simulink model "sampleModel257"  (R2021b)
settings: Solver=VariableStepAuto  StartTime=0.0  StopTime=10.0  RelTol=1e-3
undefined symbols (not defined in the file or in its folder): DiscIntNeverNeededParam, Newton, Raphson
libraries: simulink x16, slpidlib x1
settings Model: Creator=user  LastModifiedBy=user

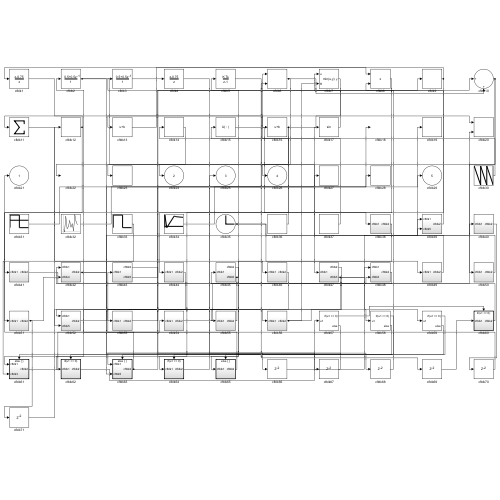
[thumbnail: Simulink's stored preview of the top-level diagram]
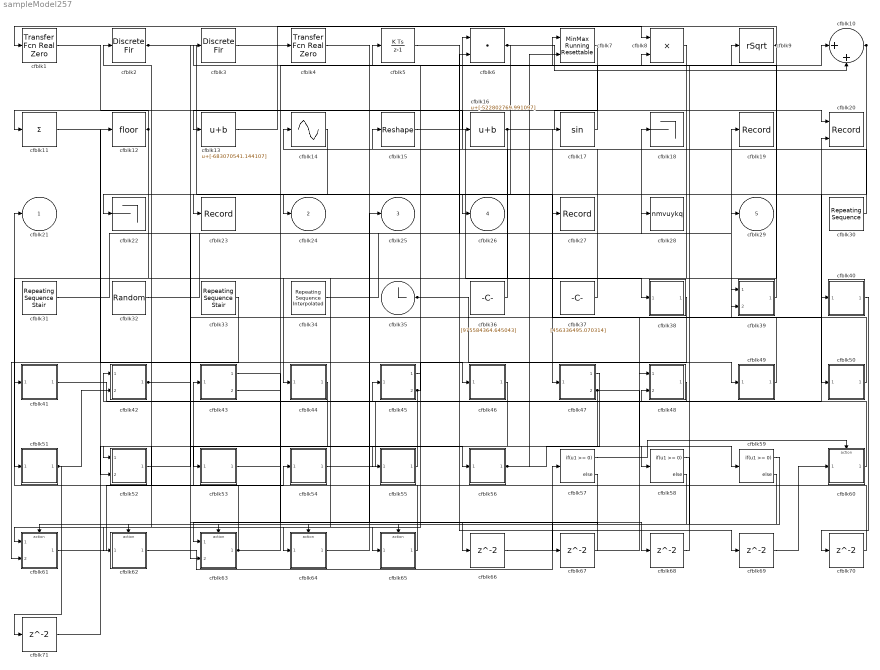
== system sampleModel257 ==
  cfblk1 : simulink/Discrete/Transfer Fcn Real Zero  ZeroZ=0.75  ICPrevInput=0.0  DoSatur=off
      settings: SourceProductBaseCode=SL
  cfblk10 : Sum  Inputs=|++
  cfblk11 : Sum  Inputs=+
  cfblk12 : Rounding
  cfblk13 : Bias  Bias=[-683070541.144107]
  cfblk14 : Sin  TimeSource=Use external signal  SampleTime=0
  cfblk15 : Reshape
  cfblk16 : Bias  Bias=[-522802769.991097]
  cfblk17 : Trigonometry
  cfblk18 : Terminator
  cfblk19 : Record  FileSettingsInternal="{\"entries\":[{\"content\":{\"excelSettings\":{\"content\":{},\"type\":\"Streamout.ExcelSettings\"}},\"type\":\"Streamout.FileSettingStorage\",\"uuid\":\"2ab1578b-86c7-4f25-b23b-f8d6f15a5c50\"}],\"packageUris\":[\"http://schema.mathworks.com/mf0/streamout_blocks/R2020a\"],\"version\":\"1.0\"}"  SignalsInternal="{\"entries\":[{\"content\":{\"signals\":[{\"content\":{\"blockPath\":[\"sampleModel257/cfblk19\"],\"channel\":[],\"dimensions\":[1],\"domain\":\"sampleModel257/cfblk19\",\"lineColor\":\"#fe330a\",\"plots\":[1],\"port\":1,\"sid\":[\"\"],\"signalID\":10619,\"signalName\":\"cfblk32\"},\"type\":\"RecordBlkView.Signal\",\"uuid\":\"c116c59d-c383-4a62-b9dd-bef188b6a92c\"}]},\"type\":\"RecordBlkView.InputSignals\",\"uuid\":\"59890f28-61aa-4252-838f-816ff403dd3c\"}],\"packageUris\":[\"http://schema.mathworks.com/mf0/streamout_blocks/R2020a\"],\"version\":\"1.0\"}"  VisualizationBindings="{\"sparklinesplugin\":{\"info\":[{\"bindingParametersList\":[],\"subplotID\":1}]}}"
  cfblk2 : DiscreteFir  SampleTime=1
  cfblk20 : Record  FileSettingsInternal="{\"entries\":[{\"content\":{\"excelSettings\":{\"content\":{},\"type\":\"Streamout.ExcelSettings\"}},\"type\":\"Streamout.FileSettingStorage\",\"uuid\":\"ddf2c5f0-8deb-4ac6-b6ac-07b526f580c7\"}],\"packageUris\":[\"http://schema.mathworks.com/mf0/streamout_blocks/R2020a\"],\"version\":\"1.0\"}"  Layout=[1 1]  SignalsInternal="{\"entries\":[{\"content\":{\"signals\":[{\"content\":{\"blockPath\":[\"sampleModel257/cfblk20\"],\"channel\":[],\"dimensions\":[1],\"domain\":\"sampleModel257/cfblk20\",\"lineColor\":\"#a2142f\",\"plots\":[1],\"port\":1,\"sid\":[\"\"],\"signalID\":10603,\"signalName\":\"cfblk16\"},\"type\":\"RecordBlkView.Signal\",\"uuid\":\"a0e00e2b-60e6-43d2-9d8d-836ea06b8f3f\"},{\"content\":{\"blockPath\":[\"sampleModel257/cfblk20\"],\"channel\":[],\"dimensions\":[1],\"domain\":\"sampleModel257/cfblk20\",\"lineColor\":\"#139fff\",\"plots\":[1],\"port\":2,\"sid\":[\"\"],\"signalID\":10607,\"signalName\":\"cfblk54\"},\"type\":\"RecordBlkView.Signal\",\"uuid\":\"187d8806-91fd-4e25-8316-ecd599589666\"}]},\"type\":\"RecordBlkView.InputSignals\",\"uuid\":\"124e2f7b-5629-4b4f-94f6-d1d15d40ce0e\"}],\"packageUris\":[\"http://schema.mathworks.com/mf0/streamout_blocks/R2020a\"],\"version\":\"1.0\"}"  VisualizationBindings="{\"xyplotplugin\":{\"info\":[{\"series\":[{\"bindingParametersList\":[{\"parameter\":\"X-Axis\",\"signalID\":10603,\"signalName\":\"cfblk16\"},{\"parameter\":\"Y-Axis\",\"signalID\":10607,\"signalName\":\"cfblk54\"}],\"seriesID\":16544}],\"subplotID\":1}]}}"  CompatibilityTag=XY
  cfblk22 : Terminator
  cfblk23 : Record  FileSettingsInternal="{\"entries\":[{\"content\":{\"excelSettings\":{\"content\":{},\"type\":\"Streamout.ExcelSettings\"}},\"type\":\"Streamout.FileSettingStorage\",\"uuid\":\"70e21285-8622-4f4c-8864-935dd75f7605\"}],\"packageUris\":[\"http://schema.mathworks.com/mf0/streamout_blocks/R2020a\"],\"version\":\"1.0\"}"  SignalsInternal="{\"entries\":[{\"content\":{\"signals\":[{\"content\":{\"blockPath\":[\"sampleModel257/cfblk23\"],\"channel\":[],\"dimensions\":[1],\"domain\":\"sampleModel257/cfblk23\",\"lineColor\":\"#ff13a6\",\"plots\":[1],\"port\":1,\"sid\":[\"\"],\"signalID\":10615,\"signalName\":\"cfblk14\"},\"type\":\"RecordBlkView.Signal\",\"uuid\":\"89a995ae-1b65-4a70-9c75-f562eec9963f\"}]},\"type\":\"RecordBlkView.InputSignals\",\"uuid\":\"2aba3f60-c205-4dbe-934f-5a1f40026660\"}],\"packageUris\":[\"http://schema.mathworks.com/mf0/streamout_blocks/R2020a\"],\"version\":\"1.0\"}"  VisualizationBindings="{\"sparklinesplugin\":{\"info\":[{\"bindingParametersList\":[],\"subplotID\":1}]}}"
  cfblk27 : Record  FileSettingsInternal="{\"entries\":[{\"content\":{\"excelSettings\":{\"content\":{},\"type\":\"Streamout.ExcelSettings\"}},\"type\":\"Streamout.FileSettingStorage\",\"uuid\":\"9b9a9fdf-4e8d-4ae3-97b2-e0004514abab\"}],\"packageUris\":[\"http://schema.mathworks.com/mf0/streamout_blocks/R2020a\"],\"version\":\"1.0\"}"  SignalsInternal="{\"entries\":[{\"content\":{\"signals\":[{\"content\":{\"blockPath\":[\"sampleModel257/cfblk27\"],\"channel\":[],\"dimensions\":[1],\"domain\":\"sampleModel257/cfblk27\",\"lineColor\":\"#64d413\",\"plots\":[1],\"port\":1,\"sid\":[\"\"],\"signalID\":10611,\"signalName\":\"cfblk63\"},\"type\":\"RecordBlkView.Signal\",\"uuid\":\"2aed3ace-228a-445a-9f27-d276254a442c\"}]},\"type\":\"RecordBlkView.InputSignals\",\"uuid\":\"1cdac96b-9a88-4913-bf08-c30701548694\"}],\"packageUris\":[\"http://schema.mathworks.com/mf0/streamout_blocks/R2020a\"],\"version\":\"1.0\"}"  VisualizationBindings="{\"sparklinesplugin\":{\"info\":[{\"bindingParametersList\":[],\"subplotID\":1}]}}"
  cfblk28 : ToWorkspace  VariableName=nmvuykq  SaveFormat=Timeseries  SampleTime=-1
  cfblk3 : DiscreteFir  SampleTime=1
  cfblk30 : simulink/Sources/Repeating Sequence  rep_seq_t=[0 2]  rep_seq_y=[196435300.380277, 69440203.193160]
  cfblk31 : simulink/Sources/Repeating Sequence Stair  OutValues=[530761793.719479, -723083426.984550]  tsamp=-1  OutMin=[]  OutMax=[]  OutDataTypeStr=double  OutputDataTypeScalingMode=double  OutDataType=fixdt(0,8)  ConRadixGroup=Best Precision: Vector-wise  OutScaling=2^-12
  cfblk32 : UniformRandomNumber  Minimum=[-9375345232.117300]  Maximum=[5045896076.837665]  Seed=[26008851.000000]  SampleTime=0.1
  cfblk33 : simulink/Sources/Repeating Sequence Stair  OutValues=[367014376.710983, 318334120.841294]  tsamp=-1  OutMin=[]  OutMax=[]  OutDataTypeStr=double  OutputDataTypeScalingMode=double  OutDataType=fixdt(0,8)  ConRadixGroup=Best Precision: Vector-wise  OutScaling=2^-12
  cfblk34 : simulink/Sources/Repeating Sequence Interpolated  OutValues=[871061618.471912, -84673037.336090, 780425661.181330, 750157126.674680, 698933664.903168]  TimeValues=[0 0.1 0.5 0.6 1].'  LookUpMeth=Use Input Nearest  tsamp=0.01  OutMin=[]  OutMax=[]  OutDataTypeStr=double  OutputDataTypeScalingMode=double  OutDataType=fixdt(0,8)  OutScaling=2^-10
  cfblk35 : Clock
  cfblk36 : Constant  Value=[975584364.645043]  SampleTime=1
  cfblk37 : Constant  Value=[456336495.070314]  SampleTime=1
  cfblk38 : Subsystem
  cfblk39 : Subsystem
  cfblk4 : simulink/Discrete/Transfer Fcn Real Zero  ZeroZ=0.75  ICPrevInput=0.0  DoSatur=off
      settings: SourceProductBaseCode=SL
  cfblk40 : Subsystem
  cfblk41 : Subsystem
  cfblk42 : Subsystem
  cfblk43 : Subsystem
  cfblk44 : Subsystem
  cfblk45 : Subsystem
  cfblk46 : Subsystem
  cfblk47 : Subsystem
  cfblk48 : Subsystem
  cfblk49 : Subsystem
  cfblk5 : DiscreteIntegrator  ICPrevOutput=DiscIntNeverNeededParam  ICPrevScaledInput=DiscIntNeverNeededParam
  cfblk50 : Subsystem
  cfblk51 : Subsystem
  cfblk52 : Subsystem
  cfblk53 : Subsystem
  cfblk54 : Subsystem
  cfblk55 : Subsystem
  cfblk56 : Subsystem
  cfblk57 : If  IfExpression=u1 >= 0  SampleTime=1
  cfblk58 : If  IfExpression=u1 >= 0  SampleTime=1
  cfblk59 : If  IfExpression=u1 >= 0  SampleTime=1
  cfblk6 : DotProduct  InputSameDT=on  OutDataTypeStr=Inherit: Inherit via internal rule
  cfblk60 : Subsystem  TreatAsAtomicUnit=on
  cfblk61 : Subsystem  TreatAsAtomicUnit=on
  cfblk62 : Subsystem  TreatAsAtomicUnit=on
  cfblk63 : Subsystem  TreatAsAtomicUnit=on
  cfblk64 : Subsystem  TreatAsAtomicUnit=on
  cfblk65 : Subsystem  TreatAsAtomicUnit=on
  cfblk{66..71} (6 alike) : Delay  SampleTime=1
  cfblk7 : simulink/Math Operations/MinMax Running Resettable  Function=min  vinit=0.0
  cfblk8 : Product
  cfblk9 : Sqrt  Operator=rSqrt  AlgorithmType=Newton-Raphson  SaturateOnIntegerOverflow=on
  cfblk21 : Outport
  cfblk24 : Outport  Port=2
  cfblk25 : Outport  Port=3
  cfblk26 : Outport  Port=4
  cfblk29 : Outport  Port=5
  wires:
  cfblk35/1 -> cfblk49/1(cfblk1), cfblk39/2(cfblk5)
  cfblk65/1(cfblk2) -> cfblk21/1
  cfblk32/1 -> cfblk19/1
  cfblk15/1 -> cfblk38/1(cfblk1)
  cfblk48/1(cfblk2) -> cfblk45/1(cfblk1)
  cfblk62/1(cfblk2) -> cfblk57/1
  cfblk34/1 -> cfblk18/1
  cfblk55/1(cfblk2) -> cfblk52/1(cfblk1)
  cfblk61/1(cfblk2) -> cfblk54/1(cfblk1)
  cfblk16/1 -> cfblk20/1, cfblk24/1, cfblk41/1(cfblk1)
  cfblk63/1(cfblk2) -> cfblk43/1(cfblk1), cfblk27/1
  cfblk12/1 -> cfblk51/1(cfblk1), cfblk11/1
  cfblk14/1 -> cfblk23/1
  cfblk30/1 -> cfblk15/1
  cfblk54/1(cfblk2) -> cfblk20/2
  cfblk8/1 -> cfblk44/1(cfblk1)
  cfblk2/1 -> cfblk47/1(cfblk1), cfblk56/1(cfblk1)
  cfblk56/1(cfblk2) -> cfblk58/1, cfblk7/2
  cfblk44/1(cfblk2) -> cfblk62/1(cfblk1)
  cfblk51/1(cfblk2) -> cfblk42/2(cfblk4), cfblk71/1
  cfblk53/1(cfblk2) -> cfblk10/1
  cfblk10/1 -> cfblk22/1, cfblk50/1(cfblk1)
  cfblk13/1 -> cfblk8/1
  cfblk45/1(cfblk2) -> cfblk61/1(cfblk1)
  cfblk33/1 -> cfblk61/2(cfblk3)
  cfblk39/1(cfblk2) -> cfblk5/1
  cfblk36/1 -> cfblk6/1
  cfblk64/1(cfblk2) -> cfblk25/1
  cfblk3/1 -> cfblk4/1
  cfblk9/1 -> cfblk64/1(cfblk1), cfblk1/1
  cfblk7/1 -> cfblk13/1
  cfblk45/2(cfblk5) -> cfblk3/1, cfblk55/1(cfblk1)
  cfblk1/1 -> cfblk16/1
  cfblk49/1(cfblk2) -> cfblk29/1
  cfblk47/1(cfblk2) -> cfblk53/1(cfblk1)
  cfblk43/2(cfblk5) -> cfblk9/1
  cfblk42/1(cfblk2) -> cfblk39/1(cfblk1), cfblk67/1
  cfblk60/1(cfblk2) -> cfblk42/1(cfblk1)
  cfblk11/1 -> cfblk46/1(cfblk1)
  cfblk52/1(cfblk2) -> cfblk28/1
  cfblk47/2(cfblk3) -> cfblk63/2(cfblk5), cfblk40/1(cfblk1), cfblk59/1
  cfblk17/1 -> cfblk7/1
  cfblk38/1(cfblk2) -> cfblk65/1(cfblk1)
  cfblk41/1(cfblk2) -> cfblk48/2(cfblk3)
  cfblk37/1 -> cfblk14/1
  cfblk31/1 -> cfblk6/2
  cfblk46/1(cfblk2) -> cfblk52/2(cfblk5)
  cfblk50/1(cfblk2) -> cfblk17/1
  cfblk6/1 -> cfblk26/1, cfblk10/2
  cfblk57/1 -> cfblk60/Action
  cfblk57/2 -> cfblk61/Action
  cfblk58/1 -> cfblk62/Action
  cfblk58/2 -> cfblk63/Action
  cfblk59/1 -> cfblk64/Action
  cfblk59/2 -> cfblk65/Action
  cfblk4/1 -> cfblk66/1
  cfblk66/1 -> cfblk48/1(cfblk1)
  cfblk67/1 -> cfblk63/1(cfblk1)
  cfblk43/1(cfblk2) -> cfblk68/1
  cfblk68/1 -> cfblk8/2
  cfblk5/1 -> cfblk69/1
  cfblk69/1 -> cfblk60/1(cfblk1)
  cfblk40/1(cfblk2) -> cfblk70/1
  cfblk70/1 -> cfblk2/1
  cfblk71/1 -> cfblk12/1

== system sampleModel257/cfblk38 ==
  cfblk1 : Inport
  cfblk3 : Sum  Inputs=-+
  cfblk2 : Outport
  wires:
  cfblk3/1 -> cfblk2/1
  cfblk1/1 -> cfblk3/1, cfblk3/2

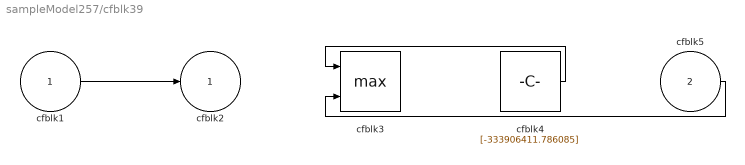
== system sampleModel257/cfblk39 ==
  cfblk1 : Inport
  cfblk5 : Inport  Port=2
  cfblk3 : MinMax  Function=max  Inputs=2
  cfblk4 : Constant  Value=[-333906411.786085]  SampleTime=1
  cfblk2 : Outport
  wires:
  cfblk1/1 -> cfblk2/1
  cfblk4/1 -> cfblk3/1
  cfblk5/1 -> cfblk3/2

== system sampleModel257/cfblk40 ==
  cfblk1 : Inport
  cfblk3 : Trigonometry
  cfblk2 : Outport
  wires:
  cfblk1/1 -> cfblk3/1
  cfblk3/1 -> cfblk2/1

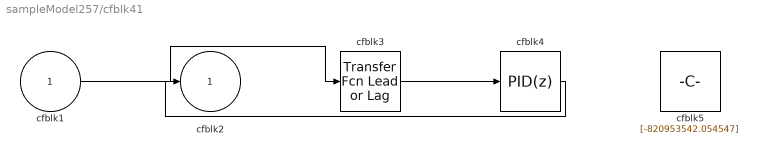
== system sampleModel257/cfblk41 ==
  cfblk1 : Inport
  cfblk3 : simulink/Discrete/Transfer Fcn Lead or Lag  PoleZ=0.95  ZeroZ=0.75  ICPrevOutput=0.0  ICPrevInput=0.0  DoSatur=off
      settings: SourceProductBaseCode=SL
  cfblk4 : slpidlib/PID Controller  Controller=PID  Form=Parallel  TimeDomain=Discrete-time  UseExternalTs=off  SampleTime=1  IntegratorMethod=Forward Euler  FilterMethod=Forward Euler  ControllerParametersSource=internal  P=1  I=1  D=0  UseFilter=on  N=100  TunerSelectOption=Transfer Function Based (PID Tuner App)  InitialConditionSource=internal  InitialConditionForIntegrator=0  InitialConditionForFilter=0  DifferentiatorICPrevScaledInput=0  ExternalReset=none  TrackingMode=off  Kt=1  LimitOutput=off  SatLimitsSource=internal  UpperSaturationLimit=inf  LowerSaturationLimit=-inf  LinearizeAsGain=off  AntiWindupMode=none  Kb=1  POutMin=[]  POutMax=[]  IOutMin=[]  IOutMax=[]  DOutMin=[]  DOutMax=[]  NOutMin=[]  NOutMax=[]  SumOutMin=[]  SumOutMax=[]  SaturationOutMin=[]  SaturationOutMax=[]  PParamMin=[]  PParamMax=[]  IParamMin=[]  IParamMax=[]  DParamMin=[]  DParamMax=[]  NParamMin=[]  NParamMax=[]  KbParamMin=[]  KbParamMax=[]  KtParamMin=[]  KtParamMax=[]  KbOutMin=[]  KbOutMax=[]  KtOutMin=[]  KtOutMax=[]  IntegratorOutMin=[]  IntegratorOutMax=[]  FilterOutMin=[]  FilterOutMax=[]  SumI1OutMin=[]  SumI1OutMax=[]  SumI2OutMin=[]  SumI2OutMax=[]  SumI3OutMin=[]  SumI3OutMax=[]  SumI4OutMin=[]  SumI4OutMax=[]  SumDOutMin=[]  SumDOutMax=[]  DifferentiatorOutMin=[]  DifferentiatorOutMax=[]  FilterDiffOutCoefMin=[]  FilterDiffOutCoefMax=[]  ReciprocalOutMin=[]  ReciprocalOutMax=[]  SumDenOutMin=[]  SumDenOutMax=[]  SumNumOutMin=[]  SumNumOutMax=[]  DivideOutMin=[]  DivideOutMax=[]  UdiffTsProdOutMin=[]  UdiffTsProdOutMax=[]  NTsProdOutMin=[]  NTsProdOutMax=[]  UintegralTsProdOutMin=[]  UintegralTsProdOutMax=[]  UngainTsProdOutMin=[]  UngainTsProdOutMax=[]  IntegratorContinuousStateAttributes=''  IntegratorStateMustResolveToSignalObject=off  IntegratorRTWStateStorageClass=Auto  FilterContinuousStateAttributes=''  FilterStateMustResolveToSignalObject=off  FilterRTWStateStorageClass=Auto  ParallelPVariant=InternalParameters  IdealPVariant=Disabled  IVariant=InternalParameters  DVariant=InternalParameters  IntegratorVariant=Discrete  SatVariant=Disabled  AWVariant=Passthrough  PCopyVariant=Disabled  TRVariant=Disabled  FdbkBlocksVariant=Forward  IdealPFdbkVariant=Disabled  SatFdbkVariant=Disabled  DerivativeFilterVariant=ForwardEulerFilter  NVariant=InternalParameters  NCopyVariant=Disabled  FilterICVariant=InternalICsFilter  IntegratorICVariant=InternalICs  ExternalResetVariant=Disabled  TRSumVariant=Passthrough  SumFdbkVariant=Disabled  SumVariant=Sum_PID  TsampFilterVariant=InternalTs  TsampNgainVariant=Passthrough  TsampIntegralVariant=Passthrough  ExternalSaturationOutDataTypeStr=Inherit: Same as second input
  cfblk5 : Constant  Value=[-820953542.054547]  SampleTime=1
  cfblk2 : Outport
  wires:
  cfblk1/1 -> cfblk3/1
  cfblk4/1 -> cfblk2/1
  cfblk3/1 -> cfblk4/1

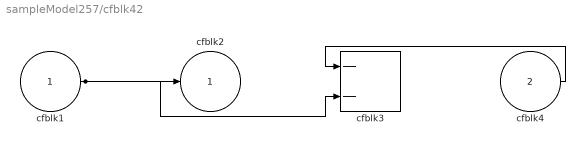
== system sampleModel257/cfblk42 ==
  cfblk1 : Inport
  cfblk4 : Inport  Port=2
  cfblk3 : Sum  Inputs=--
  cfblk2 : Outport
  wires:
  cfblk1/1 -> cfblk2/1, cfblk3/2
  cfblk4/1 -> cfblk3/1

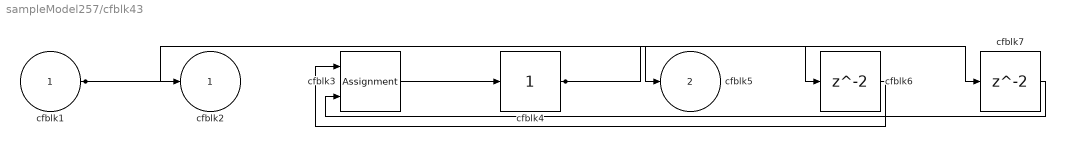
== system sampleModel257/cfblk43 ==
  cfblk1 : Inport
  cfblk3 : Assignment  DiagnosticForDimensions=Warning  IndexOptions=Index vector (dialog)  Indices=1  OutputSizes=1
  cfblk4 : simulink/Math Operations/Slider Gain  gain=1  low=0  high=2
  cfblk6 : Delay  SampleTime=1
  cfblk7 : Delay  SampleTime=1
  cfblk2 : Outport
  cfblk5 : Outport  Port=2
  wires:
  cfblk4/1 -> cfblk6/1, cfblk7/1
  cfblk3/1 -> cfblk4/1
  cfblk1/1 -> cfblk2/1, cfblk5/1
  cfblk6/1 -> cfblk3/1
  cfblk7/1 -> cfblk3/2

== system sampleModel257/cfblk44 ==
  cfblk1 : Inport
  cfblk3 : Assignment  DiagnosticForDimensions=Warning  IndexOptions=Index vector (dialog)  Indices=1  OutputSizes=1
  cfblk2 : Outport
  wires:
  cfblk1/1 -> cfblk3/1, cfblk3/2
  cfblk3/1 -> cfblk2/1

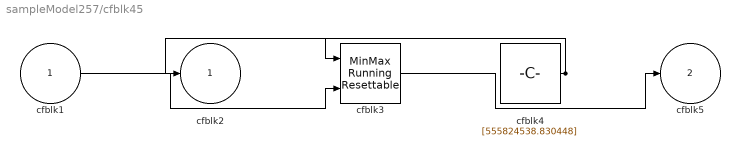
== system sampleModel257/cfblk45 ==
  cfblk1 : Inport
  cfblk3 : simulink/Math Operations/MinMax Running Resettable  Function=min  vinit=0.0
  cfblk4 : Constant  Value=[555824538.830448]  SampleTime=1
  cfblk2 : Outport
  cfblk5 : Outport  Port=2
  wires:
  cfblk4/1 -> cfblk3/1, cfblk2/1
  cfblk1/1 -> cfblk3/2
  cfblk3/1 -> cfblk5/1

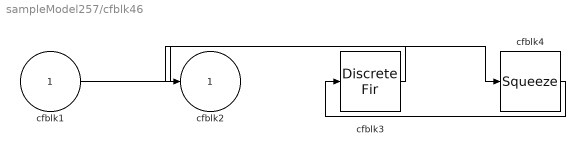
== system sampleModel257/cfblk46 ==
  cfblk1 : Inport
  cfblk3 : DiscreteFir  SampleTime=1
  cfblk4 : Squeeze
  cfblk2 : Outport
  wires:
  cfblk1/1 -> cfblk4/1
  cfblk4/1 -> cfblk3/1
  cfblk3/1 -> cfblk2/1

== system sampleModel257/cfblk47 ==
  cfblk1 : Inport
  cfblk2 : Outport
  cfblk3 : Outport  Port=2
  wires:
  cfblk1/1 -> cfblk3/1, cfblk2/1

== system sampleModel257/cfblk48 ==
  cfblk1 : Inport
  cfblk3 : Inport  Port=2
  cfblk2 : Outport
  wires:
  cfblk3/1 -> cfblk2/1

== system sampleModel257/cfblk49 ==
  cfblk1 : Inport
  cfblk3 : Sum  Inputs=+-
  cfblk4 : Bias  Bias=[31645302.167309]
  cfblk2 : Outport
  wires:
  cfblk3/1 -> cfblk2/1
  cfblk1/1 -> cfblk3/1, cfblk4/1
  cfblk4/1 -> cfblk3/2

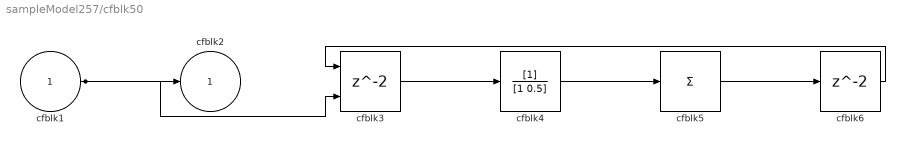
== system sampleModel257/cfblk50 ==
  cfblk1 : Inport
  cfblk3 : Delay  ShowEnablePort=on  SampleTime=1
      settings: InputPortMap=u0,e6
  cfblk4 : DiscreteFilter  SampleTime=1
  cfblk5 : Sum  Inputs=+
  cfblk6 : Delay  SampleTime=1
  cfblk2 : Outport
  wires:
  cfblk3/1 -> cfblk4/1
  cfblk1/1 -> cfblk2/1, cfblk3/2
  cfblk4/1 -> cfblk5/1
  cfblk5/1 -> cfblk6/1
  cfblk6/1 -> cfblk3/1

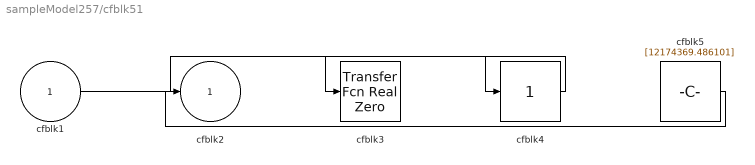
== system sampleModel257/cfblk51 ==
  cfblk1 : Inport
  cfblk3 : simulink/Discrete/Transfer Fcn Real Zero  ZeroZ=0.75  ICPrevInput=0.0  DoSatur=off
      settings: SourceProductBaseCode=SL
  cfblk4 : simulink/Math Operations/Slider Gain  gain=1  low=0  high=2
  cfblk5 : Constant  Value=[12174369.486101]  SampleTime=1
  cfblk2 : Outport
  wires:
  cfblk1/1 -> cfblk4/1
  cfblk5/1 -> cfblk2/1
  cfblk4/1 -> cfblk3/1

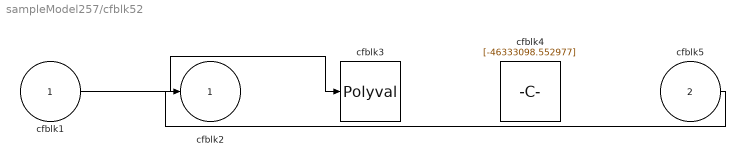
== system sampleModel257/cfblk52 ==
  cfblk1 : Inport
  cfblk5 : Inport  Port=2
  cfblk3 : Polyval  Coefs=[ +2.081618890e-019, -1.441693666e-014, +4.719686976e-010, -8.536869453e-006, +1.621573104e-001, -8.087801117e+001 ]
  cfblk4 : Constant  Value=[-46333098.552977]  SampleTime=1
  cfblk2 : Outport
  wires:
  cfblk1/1 -> cfblk3/1
  cfblk5/1 -> cfblk2/1

== system sampleModel257/cfblk53 ==
  cfblk1 : Inport
  cfblk3 : Trigonometry
  cfblk4 : simulink/Math Operations/Slider Gain  gain=1  low=0  high=2
  cfblk2 : Outport
  wires:
  cfblk4/1 -> cfblk2/1
  cfblk3/1 -> cfblk4/1
  cfblk1/1 -> cfblk3/1

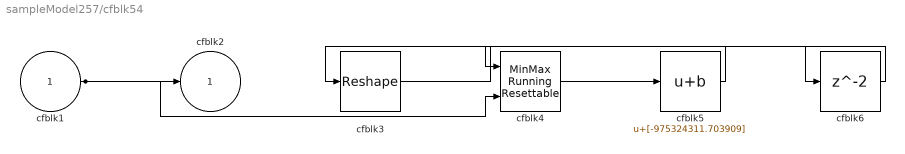
== system sampleModel257/cfblk54 ==
  cfblk1 : Inport
  cfblk3 : Reshape
  cfblk4 : simulink/Math Operations/MinMax Running Resettable  Function=min  vinit=0.0
  cfblk5 : Bias  Bias=[-975324311.703909]
  cfblk6 : Delay  SampleTime=1
  cfblk2 : Outport
  wires:
  cfblk5/1 -> cfblk3/1
  cfblk4/1 -> cfblk5/1
  cfblk1/1 -> cfblk2/1, cfblk4/2
  cfblk3/1 -> cfblk6/1
  cfblk6/1 -> cfblk4/1

== system sampleModel257/cfblk55 ==
  cfblk1 : Inport
  cfblk3 : Sum  Inputs=+
  cfblk2 : Outport
  wires:
  cfblk1/1 -> cfblk3/1
  cfblk3/1 -> cfblk2/1

== system sampleModel257/cfblk56 ==
  cfblk1 : Inport
  cfblk3 : simulink/Discrete/Difference  ICPrevInput=0.0  OutMin=[]  OutMax=[]  OutDataTypeStr=Inherit: Inherit via back propagation  OutDataType=fixdt(1, 16)  OutScaling=2^-10  DoSatur=off
  cfblk4 : Delay  DelayLengthSource=Input port  SampleTime=1
      settings: InputPortMap=u0,p1
  cfblk2 : Outport
  wires:
  cfblk1/1 -> cfblk3/1, cfblk4/1
  cfblk3/1 -> cfblk2/1, cfblk4/2

== system sampleModel257/cfblk60 ==
  cfblk1 : Inport
  Action Port : ActionPort  ActionPortLabel=if(u1 >= 0)
  cfblk3 : DiscreteIntegrator  SampleTime=-1  ICPrevOutput=DiscIntNeverNeededParam  ICPrevScaledInput=DiscIntNeverNeededParam
  cfblk2 : Outport
  wires:
  cfblk1/1 -> cfblk2/1, cfblk3/1

== system sampleModel257/cfblk61 ==
  cfblk1 : Inport
  cfblk3 : Inport  Port=2
  Action Port : ActionPort  ActionPortLabel=else
  cfblk2 : Outport
  wires:
  cfblk3/1 -> cfblk2/1

== system sampleModel257/cfblk62 ==
  cfblk1 : Inport
  Action Port : ActionPort  ActionPortLabel=if(u1 >= 0)
  cfblk3 : ComplexToRealImag
  cfblk2 : Outport
  wires:
  cfblk1/1 -> cfblk3/1
  cfblk3/1 -> cfblk2/1

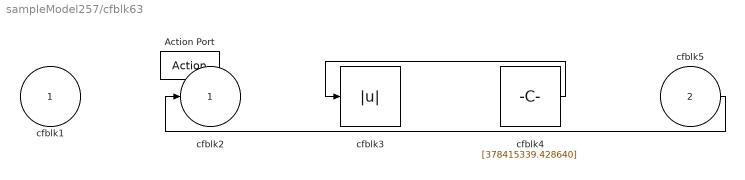
== system sampleModel257/cfblk63 ==
  cfblk1 : Inport
  cfblk5 : Inport  Port=2
  Action Port : ActionPort  ActionPortLabel=else
  cfblk3 : Abs
  cfblk4 : Constant  Value=[378415339.428640]  SampleTime=1
  cfblk2 : Outport
  wires:
  cfblk4/1 -> cfblk3/1
  cfblk5/1 -> cfblk2/1

== system sampleModel257/cfblk64 ==
  cfblk1 : Inport
  Action Port : ActionPort  ActionPortLabel=if(u1 >= 0)
  cfblk3 : ComplexToRealImag
  cfblk2 : Outport
  wires:
  cfblk1/1 -> cfblk3/1
  cfblk3/1 -> cfblk2/1

== system sampleModel257/cfblk65 ==
  cfblk1 : Inport
  Action Port : ActionPort  ActionPortLabel=else
  cfblk3 : simulink/Discrete/Transfer Fcn First Order  PoleZ=0.95  ICPrevOutput=0.0  DoSatur=off
  cfblk2 : Outport
  wires:
  cfblk1/1 -> cfblk3/1
  cfblk3/1 -> cfblk2/1
